simulink model "example_tcp"  (R2022b)
settings: Solver=FixedStepAuto  StartTime=0.0  StopTime=1000.0  FixedStep=0.2  RelTol=1e-3
libraries: slrealtimeiplib x2, instrumentlib x2
settings Model: Creator=33093  LastModifiedBy=33093

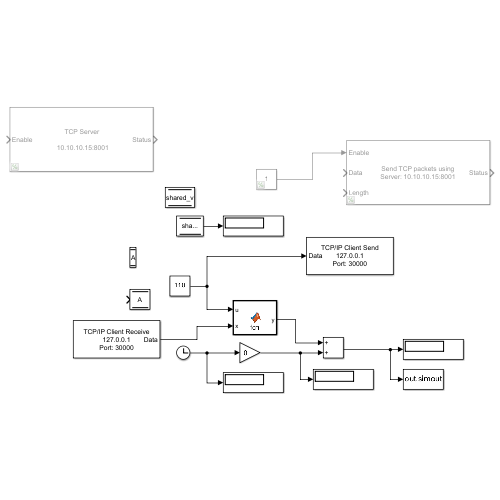
[thumbnail: Simulink's stored preview of the top-level diagram]
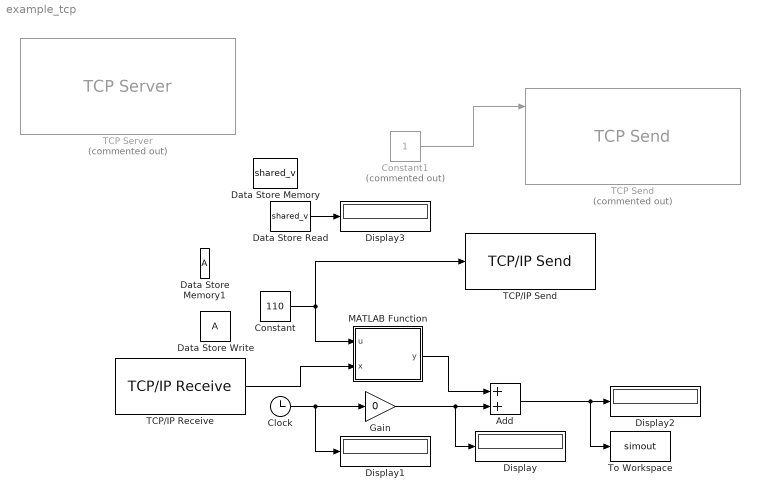
== system example_tcp ==
  Add : Sum
  Clock : Clock
  Constant : Constant  Value=110
  Constant1 : Constant  Commented=on
  Data Store Memory : DataStoreMemory  DataStoreName=shared_v  WriteAfterWriteMsg=warning  InitialValue=1  ShowAdditionalParam=off  OutDataTypeStr=double
  Data Store Memory1 : DataStoreMemory  WriteAfterWriteMsg=warning  ShowAdditionalParam=off
  Data Store Read : DataStoreRead  DataStoreName=shared_v  DataStoreElements=shared_v  IndexOptions=Index vector (dialog)  Indices=1  OutputSizes=1
  Data Store Write : DataStoreWrite  IndexOptions=Index vector (dialog)  Indices=1  OutputSizes=1
  Display{,1..3} (4 alike) : Display
  Gain : Gain  Gain=0
  MATLAB Function : MATLAB Function  TreatAsAtomicUnit=on
  TCP Send : slrealtimeiplib/TCP Send  Commented=on  socketAddPortVal=Server: 10.10.10.15:8001  sampleTime=-1
  TCP Server : slrealtimeiplib/TCP Server  Priority=-1  Commented=on  useHostTargetConn=off  serverAddress=10.10.10.15  serverPort=8001
  TCP/IP Receive : instrumentlib/TCP//IP Receive  Host=127.0.0.1  Port=30000  DataSize=[ 1, 1 ]  DataType=double  ASCIIFormatting=%f  Terminator=LF  CustomTerminator=10  ByteOrder=big-endian  EnableBlockingMode=on  Timeout=10  SampleTime=0.2  SimulateUsing=Interpreted execution
  TCP/IP Send : instrumentlib/TCP//IP Send  Host=127.0.0.1  Port=30000  ByteOrder=little-endian  EnableBlockingMode=on  Timeout=10  TransferDelay=on  SimulateUsing=Interpreted execution
  To Workspace : ToWorkspace  VariableName=simout  SampleTime=-1
  wires:
  Add/1 -> Display2/1, To Workspace/1
  Constant/1 -> TCP/IP Send/1, MATLAB Function/1(u)
  Data Store Read/1 -> Display3/1
  Clock/1 -> Gain/1, Display1/1
  MATLAB Function/1(y) -> Add/1
  Gain/1 -> Add/2, Display/1
  TCP/IP Receive/1 -> MATLAB Function/2(x)
  Constant1/1 -> TCP Send/1

== matlab function example_tcp/MATLAB Function ==
  data: u input; y output; shared_v data_store_memory; x input
function y = fcn(u, x)
y = x;
end
